simulink model "DynamicSystemModel"  (R2017a)
settings: Solver=ode45  StartTime=0.0  StopTime=24  RelTol=1e-3
PreLoadFcn:
  | load('ex_househeat_measured_data.mat')
model workspace (MAT data in the model file):
  M_heater_air = 3600
  R_equivalent = 4.329e-07
  T_heater = 50
  T_roomIC = 20
  c_air = 1005.4
  m_room_air = 1470
settings Model: Creator=Hyperion  LastModifiedBy=Hyperion
settings DataIOCC: ExternalInput=Sheet1.getElement(1),Sheet1.getElement(2)  LoadExternalInput=on  SaveOutput=off  InspectSignalLogs=on  SaveTime=off
settings OptimizationCC: BlockReduction=off

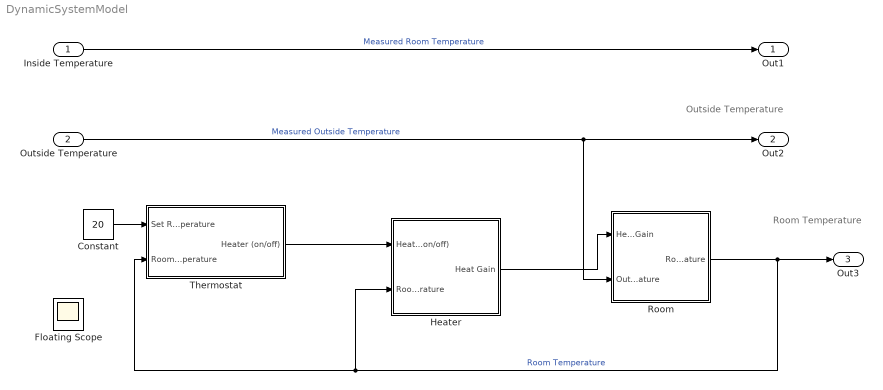
== system DynamicSystemModel ==
  note: Outside
      | Temperature
  note: Room
      | Temperature
  Inside Temperature : Inport
  Outside Temperature : Inport  Port=2  Unit=°C
  Constant : Constant  Value=20
  Floating Scope : Scope
      settings: Floating=on
  Heater : Subsystem
  Room : Subsystem
  Thermostat : Subsystem
  Out1 : Outport
  Out2 : Outport  Port=2  Unit=°C
  Out3 : Outport  Port=3  Unit=°C
  wires:
  Thermostat/1(Heater (on/off)) -> Heater/1(Heater (on/off))
  Room/1(Room Temperature) -> Heater/2(Room Temperature), Thermostat/2(Room Temperature), Out3/1  "Room Temperature"
  Heater/1(Heat Gain) -> Room/1(Heat Gain)
  Outside Temperature/1 -> Room/2(Outside Temperature), Out2/1  "Measured Outside Temperature"
  Constant/1 -> Thermostat/1(Set Room Temperature)
  Inside Temperature/1 -> Out1/1  "Measured Room Temperature"

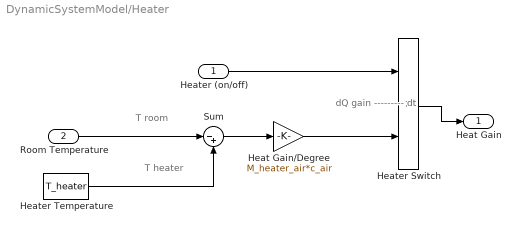
== system DynamicSystemModel/Heater ==
  note: dQ gain
      | ---------
      | dt
  note: T heater
  note: T room
  Heater (on/off) : Inport
  Room Temperature : Inport  Port=2  Unit=°C
  Heat Gain/Degree : Gain  Gain=M_heater_air*c_air
  Heater Switch : Product
  Heater Temperature : Constant  Value=T_heater
  Sum : Sum  Inputs=|-+
  Heat Gain : Outport  Unit=joule/h
  wires:
  Heater Temperature/1 -> Sum/2
  Room Temperature/1 -> Sum/1
  Sum/1 -> Heat Gain/Degree/1
  Heater (on/off)/1 -> Heater Switch/1
  Heater Switch/1 -> Heat Gain/1
  Heat Gain/Degree/1 -> Heater Switch/2

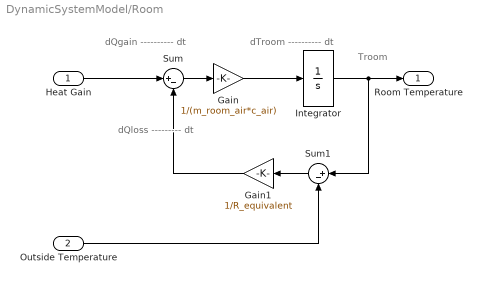
== system DynamicSystemModel/Room ==
  note: Troom
  note: dTroom
      | ----------
      |     dt
  note: dQloss
      | ---------
      |    dt
  note: dQgain
      | ----------
      |    dt
  Heat Gain : Inport
  Outside Temperature : Inport  Port=2
  Gain : Gain  Gain=1/(m_room_air*c_air)
  Gain1 : Gain  Gain=1/R_equivalent
  Integrator : Integrator  InitialCondition=T_roomIC
  Sum : Sum  Inputs=|+-
  Sum1 : Sum  Inputs=|+-
  Room Temperature : Outport
  wires:
  Heat Gain/1 -> Sum/1
  Gain1/1 -> Sum/2
  Sum/1 -> Gain/1
  Gain/1 -> Integrator/1
  Integrator/1 -> Sum1/1, Room Temperature/1
  Sum1/1 -> Gain1/1
  Outside Temperature/1 -> Sum1/2

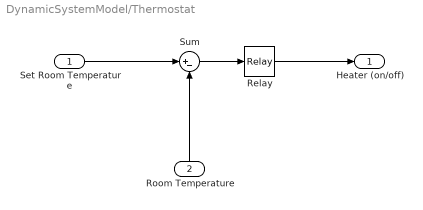
== system DynamicSystemModel/Thermostat ==
  Set Room Temperature : Inport
  Room Temperature : Inport  Port=2
  Relay : Relay  OnSwitchValue=0  OffSwitchValue=-5
  Sum : Sum  Inputs=|+-
  Heater (on/off) : Outport
  wires:
  Sum/1 -> Relay/1
  Relay/1 -> Heater (on/off)/1
  Set Room Temperature/1 -> Sum/1
  Room Temperature/1 -> Sum/2
